simulink model "EvitaParedes"  (R2023b)
settings: Solver=VariableStepAuto  StartTime=0.0  StopTime=10.0  RelTol=1e-3
settings Model: Creator=Carlos  LastModifiedBy=Carlos

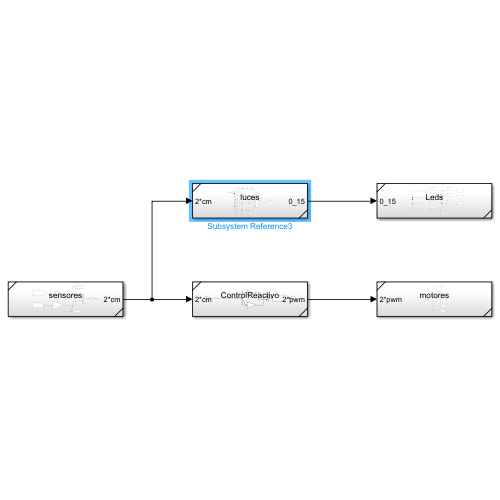
[thumbnail: Simulink's stored preview of the top-level diagram]
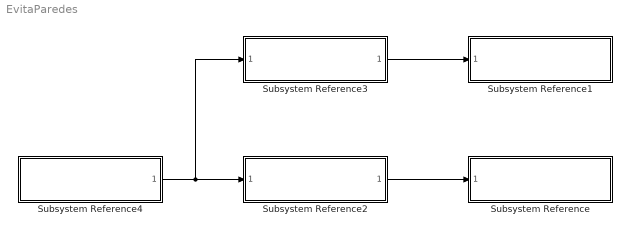
== system EvitaParedes ==
  Subsystem Reference : Subsystem  ReferencedSubsystem=motores
  Subsystem Reference1 : Subsystem  ReferencedSubsystem=Leds
  Subsystem Reference2 : Subsystem  ReferencedSubsystem=ControlReactivo
  Subsystem Reference3 : Subsystem  ReferencedSubsystem=luces
  Subsystem Reference4 : Subsystem  ReferencedSubsystem=sensores
  wires:
  Subsystem Reference2/1 -> Subsystem Reference/1
  Subsystem Reference3/1 -> Subsystem Reference1/1
  Subsystem Reference4/1 -> Subsystem Reference3/1, Subsystem Reference2/1
